simulink model "PID_Control"  (R2021b)
settings: Solver=VariableStepAuto  StartTime=0.0  StopTime=10.0  RelTol=1e-3
values from neighbouring files (symbols this model uses):
  Kd = 1    [Task1_input_value.m]
  Ki = 13    [Task1_input_value.m]
  Kp = 300    [Task1_input_value.m]
  Ts = 0.01    [Task1_input_value.m]
settings Model: Creator=vinod  LastModifiedBy=vinod

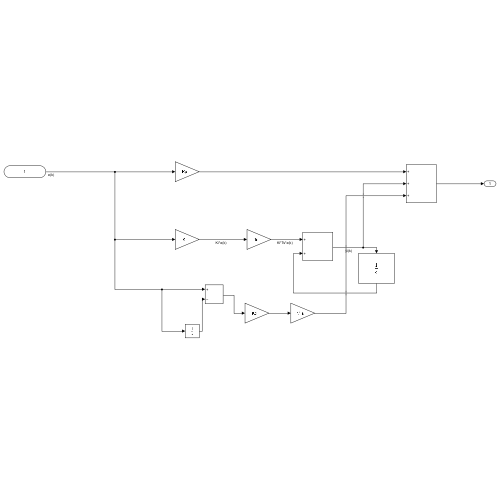
[thumbnail: Simulink's stored preview of the top-level diagram]
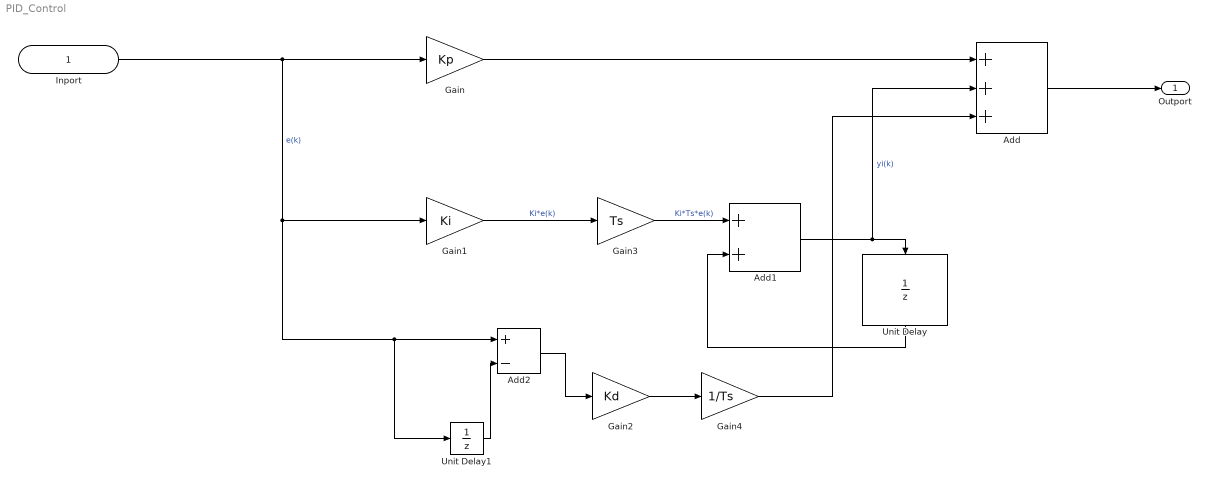
== system PID_Control ==
  Inport : Inport  OutDataTypeStr=double  PortDimensions=1  SampleTime=Ts
  Add : Sum  Inputs=+++
  Add1 : Sum
  Add2 : Sum  Inputs=+-
  Gain : Gain  Gain=Kp
  Gain1 : Gain  Gain=Ki
  Gain2 : Gain  Gain=Kd
  Gain3 : Gain  Gain=Ts
  Gain4 : Gain  Gain=1/Ts
  Unit Delay : UnitDelay  SampleTime=-1  HasFrameUpgradeWarning=on
  Unit Delay1 : UnitDelay  SampleTime=-1  HasFrameUpgradeWarning=on
  Outport : Outport  OutDataTypeStr=double  PortDimensions=1  SampleTime=Ts
  wires:
  Gain4/1 -> Add/3
  Add2/1 -> Gain2/1
  Gain/1 -> Add/1
  Gain2/1 -> Gain4/1
  Add/1 -> Outport/1
  Inport/1 -> Add2/1, Unit Delay1/1, Gain1/1, Gain/1  "e(k)"
  Add1/1 -> Add/2, Unit Delay/1  "yi(k)"
  Gain3/1 -> Add1/1  "Ki*Ts*e(k)"
  Gain1/1 -> Gain3/1  "Ki*e(k)"
  Unit Delay/1 -> Add1/2
  Unit Delay1/1 -> Add2/2
